simulink model "Simulation_With_PreviousData"  (R2020b)
settings: Solver=ode15s  StartTime=0.0  StopTime=10  RelTol=1e-3
undefined symbols (not defined in the file): X, Y, Z
libraries: sm_lib x71, nesl_utility x13
(part 2 of 2)

== matlab function Simulation_With_PreviousData/angular velocity lk ==
  data: x input; y output
function y = fcn(x)

       
       a1 =       13.68  ;
       b1 =      -8.087  ;
       a2 =      -7.783  ;
       b2 =       3.265  ;
       a3 =       -4.76  ;
       b3 =       13.73  ;
       a4 =      -4.566  ;
       b4 =        2.01  ;
       w =       1.944  ;



y = a1*w*sin(w*x) - 2*b2*w*cos(2*w*x) - 3*b3*w*cos(3*w*x) - 4*b4*w*cos(4*w*x) - b1*w*cos(w*x) + 2*a2*w*sin(2*w*x) + 3*a3*w*sin(3*w*x) + 4*a4*w*sin(4*w*x);

== matlab function Simulation_With_PreviousData/angle la ==
  data: x input; y output
function y = fcn(x)

       a0 =      -3.553  ;
       a1 =      -7.876  ;
       b1 =      -2.493  ;
       a2 =       -8.22  ;
       b2 =      -3.326  ;
       w =       2.689  ;

y =  a0 + a1*cos(x*w) + b1*sin(x*w) + ...
               a2*cos(2*x*w) + b2*sin(2*x*w);

== matlab function Simulation_With_PreviousData/angular acceleration la ==
  data: x input; y output
function y = fcn(x)

       a1 =      -7.876  ;
       b1 =      -2.493  ;
       a2 =       -8.22  ;
       b2 =      -3.326  ;
       w =       2.689  ;



y=- a1*w^2*cos(w*x) - 4*a2*w^2*cos(2*w*x) - b1*w^2*sin(w*x) - 4*b2*w^2*sin(2*w*x);

== matlab function Simulation_With_PreviousData/angular velocity la ==
  data: x input; y output
function y = fcn(x)

       
       a1 =      -7.876  ;
       b1 =      -2.493  ;
       a2 =       -8.22  ;
       b2 =      -3.326  ;
       w =       2.689  ;



y = b1*w*cos(w*x) + 2*b2*w*cos(2*w*x) - a1*w*sin(w*x) - 2*a2*w*sin(2*w*x);

== matlab function Simulation_With_PreviousData/angular acceleration rk1 ==
  data: x input; y output
function y = fcn(x)

       a1 =      -3.531  ;
       b1 =      -16.66 ;
       a2 =      -8.844  ;
       b2 =       9.965  ;
       a3 =      -0.609 ;
       b3 =       3.416  ;
       a4 =     0.08159  ;
       b4 =     -0.1367 ;
       w =       3.082  ;



y=a1*w^2*cos(w*x) + 4*a2*w^2*cos(2*w*x) + 9*a3*w^2*cos(3*w*x) + 16*a4*w^2*cos(4*w*x) + b1*w^2*sin(w*x) + 4*b2*w^2*sin(2*w*x) + 9*b3*w^2*sin(3*w*x) + 16*b4*w^2*sin(4*w*x);

== matlab function Simulation_With_PreviousData/angle rh ==
  data: x input; y output
function y = fcn(x)

       a0 =       7.547  ;
       a1 =       23.09  ;
       b1 =      -8.588 ;
       a2 =      -3.746  ;
       b2 =      0.8751  ;
       a3 =     -0.2391  ;
       b3 =       1.835  ;
       a4 =      0.1478  ;
       b4 =    -0.03261  ;
       w =       3.014  ;

y = a0 + a1*cos(x*w) + b1*sin(x*w) + ...
               a2*cos(2*x*w) + b2*sin(2*x*w) + a3*cos(3*x*w) + b3*sin(3*x*w) + ...
               a4*cos(4*x*w) + b4*sin(4*x*w);

== matlab function Simulation_With_PreviousData/angular acceleration rh ==
  data: x input; y output
function y = fcn(x)

       a1 =       23.09  ;
       b1 =      -8.588 ;
       a2 =      -3.746  ;
       b2 =      0.8751  ;
       a3 =     -0.2391  ;
       b3 =       1.835  ;
       a4 =      0.1478  ;
       b4 =    -0.03261  ;
       w =       3.014  ;



y = - a1*w^2*cos(w*x) - 4*a2*w^2*cos(2*w*x) - 9*a3*w^2*cos(3*w*x) - 16*a4*w^2*cos(4*w*x) - b1*w^2*sin(w*x) - 4*b2*w^2*sin(2*w*x) - 9*b3*w^2*sin(3*w*x) - 16*b4*w^2*sin(4*w*x);

== matlab function Simulation_With_PreviousData/angle rk ==
  data: x input; y output
function y = fcn(x)

       a0 =       16.67  ;
       a1 =      -3.531  ;
       b1 =      -16.66 ;
       a2 =      -8.844  ;
       b2 =       9.965  ;
       a3 =      -0.609 ;
       b3 =       3.416  ;
       a4 =     0.08159  ;
       b4 =     -0.1367 ;
       w =       3.082  ;

y = -(a0 + a1*cos(x*w) + b1*sin(x*w) + ...
               a2*cos(2*x*w) + b2*sin(2*x*w) + a3*cos(3*x*w) + b3*sin(3*x*w) + ...
               a4*cos(4*x*w) + b4*sin(4*x*w));

== matlab function Simulation_With_PreviousData/angular velocity rh ==
  data: x input; y output
function y = fcn(x)

       
       a1 =       23.09  ;
       b1 =      -8.588 ;
       a2 =      -3.746  ;
       b2 =      0.8751  ;
       a3 =     -0.2391  ;
       b3 =       1.835  ;
       a4 =      0.1478  ;
       b4 =    -0.03261  ;
       w =       3.014  ;



y = b1*w*cos(w*x) + 2*b2*w*cos(2*w*x) + 3*b3*w*cos(3*w*x) + 4*b4*w*cos(4*w*x) - a1*w*sin(w*x) - 2*a2*w*sin(2*w*x) - 3*a3*w*sin(3*w*x) - 4*a4*w*sin(4*w*x);

== matlab function Simulation_With_PreviousData/angular velocity rk ==
  data: x input; y output
function y = fcn(x)

       
       a1 =      -3.531  ;
       b1 =      -16.66 ;
       a2 =      -8.844  ;
       b2 =       9.965  ;
       a3 =      -0.609 ;
       b3 =       3.416  ;
       a4 =     0.08159  ;
       b4 =     -0.1367 ;
       w =       3.082  ;



y=a1*w*sin(w*x) - 2*b2*w*cos(2*w*x) - 3*b3*w*cos(3*w*x) - 4*b4*w*cos(4*w*x) - b1*w*cos(w*x) + 2*a2*w*sin(2*w*x) + 3*a3*w*sin(3*w*x) + 4*a4*w*sin(4*w*x);

== matlab function Simulation_With_PreviousData/angular acceleration ra ==
  data: x input; y output
function y = fcn(x)

       a1 =       4.529  ;
       b1 =       5.133 ;
       a2 =      -1.302  ;
       b2 =      -9.381  ;
       a3 =      -1.241  ;
       b3 =       2.598 ;
       a4 =      0.8422  ;
       b4 =      -2.712  ;
       w =       3.062  ;



y = - a1*w^2*cos(w*x) - 4*a2*w^2*cos(2*w*x) - 9*a3*w^2*cos(3*w*x) - 16*a4*w^2*cos(4*w*x) - b1*w^2*sin(w*x) - 4*b2*w^2*sin(2*w*x) - 9*b3*w^2*sin(3*w*x) - 16*b4*w^2*sin(4*w*x);

== matlab function Simulation_With_PreviousData/angular velocity ra ==
  data: x input; y output
function y = fcn(x)

       
       a1 =       4.529  ;
       b1 =       5.133 ;
       a2 =      -1.302  ;
       b2 =      -9.381  ;
       a3 =      -1.241  ;
       b3 =       2.598 ;
       a4 =      0.8422  ;
       b4 =      -2.712  ;
       w =       3.062  ;



y = b1*w*cos(w*x) + 2*b2*w*cos(2*w*x) + 3*b3*w*cos(3*w*x) + 4*b4*w*cos(4*w*x) - a1*w*sin(w*x) - 2*a2*w*sin(2*w*x) - 3*a3*w*sin(3*w*x) - 4*a4*w*sin(4*w*x);

== matlab function Simulation_With_PreviousData/angle ra ==
  data: x input; y output
function y = fcn(x)

      a0 =      -2.739  ;
       a1 =       4.529  ;
       b1 =       5.133 ;
       a2 =      -1.302  ;
       b2 =      -9.381  ;
       a3 =      -1.241  ;
       b3 =       2.598 ;
       a4 =      0.8422  ;
       b4 =      -2.712  ;
       w =       3.062  ;

y = a0 + a1*cos(x*w) + b1*sin(x*w) + ...
               a2*cos(2*x*w) + b2*sin(2*x*w) + a3*cos(3*x*w) + b3*sin(3*x*w) + ...
               a4*cos(4*x*w) + b4*sin(4*x*w);

== matlab function Simulation_With_PreviousData/angle lh ==
  data: x input; y output
function y = fcn(x)

       a0 =       8.491  ;
       a1 =      -21.68  ;
       b1 =       10.46  ;
       a2 =      -4.006  ;
       b2 =       2.165  ;
       a3 =       -0.54  ;
       b3 =      -1.482  ;
       a4 =    -0.05594  ;
       b4 =   -0.006959  ;
       w =       3.084  ;

y = a0 + a1*cos(x*w) + b1*sin(x*w) + ...
               a2*cos(2*x*w) + b2*sin(2*x*w) + a3*cos(3*x*w) + b3*sin(3*x*w) + ...
               a4*cos(4*x*w) + b4*sin(4*x*w);

== matlab function Simulation_With_PreviousData/angular acceleration lh ==
  data: x input; y output
function y = fcn(x)

       a1 =      -21.68  ;
       b1 =       10.46  ;
       a2 =      -4.006  ;
       b2 =       2.165  ;
       a3 =       -0.54  ;
       b3 =      -1.482  ;
       a4 =    -0.05594  ;
       b4 =   -0.006959  ;
       w =       3.084  ;



y = - a1*w^2*cos(w*x) - 4*a2*w^2*cos(2*w*x) - 9*a3*w^2*cos(3*w*x) - 16*a4*w^2*cos(4*w*x) - b1*w^2*sin(w*x) - 4*b2*w^2*sin(2*w*x) - 9*b3*w^2*sin(3*w*x) - 16*b4*w^2*sin(4*w*x);

== matlab function Simulation_With_PreviousData/angular velocity lh ==
  data: x input; y output
function y = fcn(x)

       
       a1 =      -21.68  ;
       b1 =       10.46  ;
       a2 =      -4.006  ;
       b2 =       2.165  ;
       a3 =       -0.54  ;
       b3 =      -1.482  ;
       a4 =    -0.05594  ;
       b4 =   -0.006959  ;
       w =       3.084  ;



y = b1*w*cos(w*x) + 2*b2*w*cos(2*w*x) + 3*b3*w*cos(3*w*x) + 4*b4*w*cos(4*w*x) - a1*w*sin(w*x) - 2*a2*w*sin(2*w*x) - 3*a3*w*sin(3*w*x) - 4*a4*w*sin(4*w*x);

== matlab function Simulation_With_PreviousData/angle lk ==
  data: x input; y output
function y = fcn(x)

       a0 =       21.96  ;
       a1 =       13.68  ;
       b1 =      -8.087  ;
       a2 =      -7.783  ;
       b2 =       3.265  ;
       a3 =       -4.76  ;
       b3 =       13.73  ;
       a4 =      -4.566  ;
       b4 =        2.01  ;
       w =       1.944  ;

y = -(a0 + a1*cos(x*w) + b1*sin(x*w) + ...
               a2*cos(2*x*w) + b2*sin(2*x*w) + a3*cos(3*x*w) + b3*sin(3*x*w) + ...
               a4*cos(4*x*w) + b4*sin(4*x*w));

== matlab function Simulation_With_PreviousData/angular acceleration lk ==
  data: x input; y output
function y = fcn(x)

       a1 =       13.68  ;
       b1 =      -8.087  ;
       a2 =      -7.783  ;
       b2 =       3.265  ;
       a3 =       -4.76  ;
       b3 =       13.73  ;
       a4 =      -4.566  ;
       b4 =        2.01  ;
       w =       1.944  ;



y = a1*w^2*cos(w*x) + 4*a2*w^2*cos(2*w*x) + 9*a3*w^2*cos(3*w*x) + 16*a4*w^2*cos(4*w*x) + b1*w^2*sin(w*x) + 4*b2*w^2*sin(2*w*x) + 9*b3*w^2*sin(3*w*x) + 16*b4*w^2*sin(4*w*x);
